simulink model "disturbances_test"  (R2016b)
settings: Solver=VariableStepAuto  StartTime=0.0  StopTime=5400  RelTol=1e-3
values from neighbouring files (symbols this model uses):
  fsw_params = init_fsw_params()    [init_disturbances_test.m]    (also in init_environment_test.m)
undefined symbols (not defined in the file or in its folder): sim_params
libraries: environment_lib x2, aerolibutil x2, vrlib x1, time_conversions_lib x1, eci_2_ecef_lib x1, sgp4_lib_fsw x1, teme_2_eci_lib x1
settings Model: Creator=taylorreynolds  LastModifiedBy=taylorreynolds

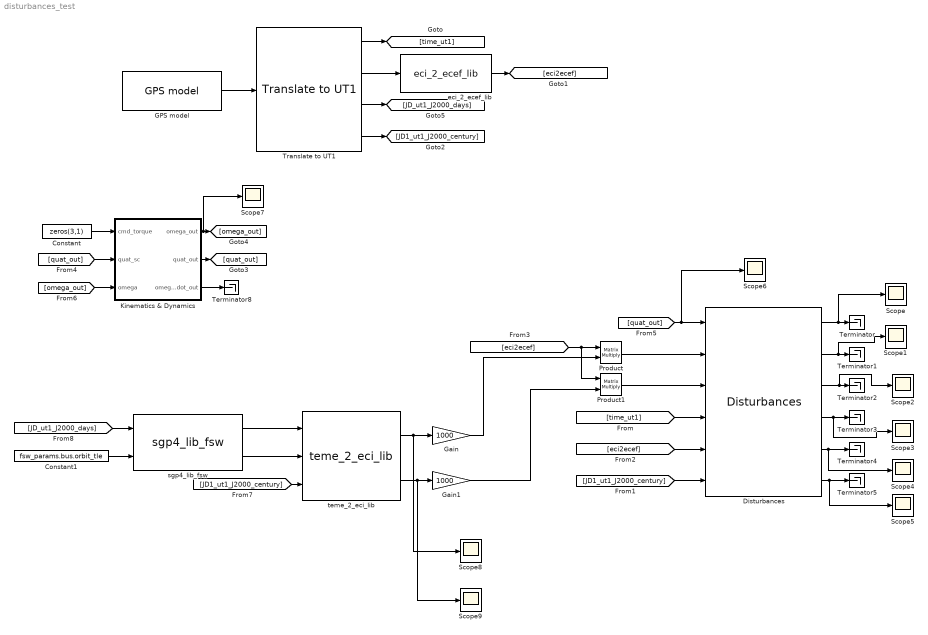
== system disturbances_test ==
  Constant : Constant  Value=zeros(3,1)
  Constant1 : Constant  Value=fsw_params.bus.orbit_tle
  Disturbances : environment_lib/Environment/Disturbances
  GPS model : environment_lib/Environment/GPS model
  Gain : Gain  Gain=1000
  Gain1 : Gain  Gain=1000
  Kinematics & Dynamics : Subsystem
  Product : Product  Multiplication=Matrix(*)
  Product1 : Product  Multiplication=Matrix(*)
  Scope{,1..9} (10 alike) : Scope
  Terminator{,1..5,8} (7 alike) : Terminator
  Translate to UT1 : time_conversions_lib/Translate to UT1
  eci_2_ecef_lib : eci_2_ecef_lib/eci_2_ecef_lib
  sgp4_lib_fsw : sgp4_lib_fsw/sgp4_lib_fsw
  teme_2_eci_lib : teme_2_eci_lib/teme_2_eci_lib
  wires:
  GPS model/1 -> Translate to UT1/1
  Translate to UT1/2 -> eci_2_ecef_lib/1
  Translate to UT1/1 -> [time_ut1]
  [time_ut1] -> Disturbances/4
  eci_2_ecef_lib/1 -> [eci2ecef]
  Translate to UT1/4 -> [JD1_ut1_J2000_century]
  [JD1_ut1_J2000_century] -> Disturbances/6
  [eci2ecef] -> Disturbances/5
  Gain/1 -> Product/2
  Product/1 -> Disturbances/2
  Product1/1 -> Disturbances/3
  Gain1/1 -> Product1/2
  [eci2ecef] -> Product1/1, Product/1
  Disturbances/1 -> Scope/1, Terminator/1
  Disturbances/2 -> Scope1/1, Terminator1/1
  Disturbances/3 -> Scope2/1, Terminator2/1
  Disturbances/4 -> Scope3/1, Terminator3/1
  Disturbances/5 -> Terminator4/1, Scope4/1
  Disturbances/6 -> Scope5/1, Terminator5/1
  Translate to UT1/3 -> [JD_ut1_J2000_days]
  Constant/1 -> Kinematics & Dynamics/1(cmd_torque)
  Kinematics & Dynamics/1(omega_out) -> Scope7/1, [omega_out]
  Kinematics & Dynamics/3(omega_dot_out) -> Terminator8/1
  Kinematics & Dynamics/2(quat_out) -> [quat_out]
  [quat_out] -> Scope6/1, Disturbances/1
  [quat_out] -> Kinematics & Dynamics/2(quat_sc)
  [omega_out] -> Kinematics & Dynamics/3(omega)
  Constant1/1 -> sgp4_lib_fsw/2
  teme_2_eci_lib/2 -> Scope9/1, Gain1/1
  teme_2_eci_lib/1 -> Scope8/1, Gain/1
  sgp4_lib_fsw/1 -> teme_2_eci_lib/1
  sgp4_lib_fsw/2 -> teme_2_eci_lib/2
  [JD1_ut1_J2000_century] -> teme_2_eci_lib/3
  [JD_ut1_J2000_days] -> sgp4_lib_fsw/1

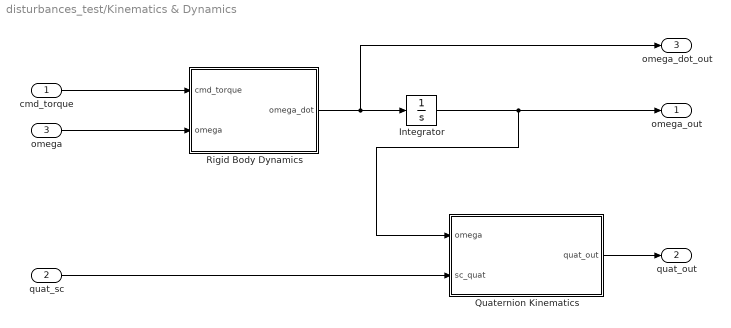
== system disturbances_test/Kinematics & Dynamics ==
  cmd_torque : Inport
  quat_sc : Inport  Port=2
  omega : Inport  Port=3
  Integrator : Integrator  InitialCondition=sim_params.dynamics.ic.rate_init
  Quaternion Kinematics : Subsystem
  Rigid Body Dynamics : Subsystem
  omega_out : Outport
  quat_out : Outport  Port=2
  omega_dot_out : Outport  Port=3
  wires:
  Rigid Body Dynamics/1(omega_dot) -> omega_dot_out/1, Integrator/1
  Integrator/1 -> Quaternion Kinematics/1(omega), omega_out/1
  cmd_torque/1 -> Rigid Body Dynamics/1(cmd_torque)
  omega/1 -> Rigid Body Dynamics/2(omega)
  Quaternion Kinematics/1(quat_out) -> quat_out/1
  quat_sc/1 -> Quaternion Kinematics/2(sc_quat)

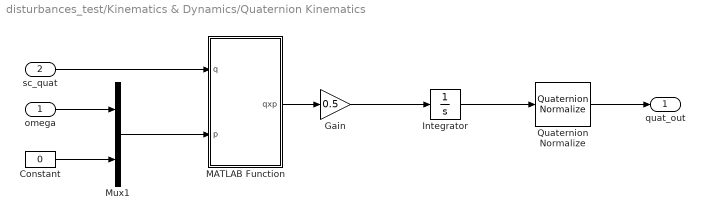
== system disturbances_test/Kinematics & Dynamics/Quaternion Kinematics ==
  omega : Inport
  sc_quat : Inport  Port=2
  Constant : Constant  Value=0
  Gain : Gain  Gain=0.5
  Integrator : Integrator  InitialCondition=sim_params.dynamics.ic.quat_init
  MATLAB Function : MATLAB Function  TreatAsAtomicUnit=on
  Mux1 : Mux  Inputs=[3 1]
  Quaternion Normalize : aerolibutil/Quaternion Normalize
  quat_out : Outport
  wires:
  Mux1/1 -> MATLAB Function/2(p)
  MATLAB Function/1(qxp) -> Gain/1
  Gain/1 -> Integrator/1
  Integrator/1 -> Quaternion Normalize/1
  Quaternion Normalize/1 -> quat_out/1
  sc_quat/1 -> MATLAB Function/1(q)
  omega/1 -> Mux1/1
  Constant/1 -> Mux1/2

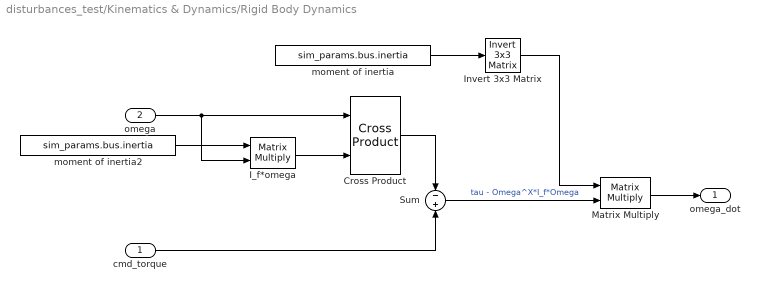
== system disturbances_test/Kinematics & Dynamics/Rigid Body Dynamics ==
  cmd_torque : Inport
  omega : Inport  Port=2
  Cross Product : vrlib/Utilities/Cross Product
  I_f*omega : Product  Multiplication=Matrix(*)
  Invert 3x3 Matrix : aerolibutil/Invert  3x3 Matrix
  "Matrix Multiply " : Product  Multiplication=Matrix(*)
  Sum : Sum  Inputs=-+
  moment of inertia : Constant  Value=sim_params.bus.inertia
  moment of inertia2 : Constant  Value=sim_params.bus.inertia
  omega_dot : Outport
  wires:
  omega/1 -> I_f*omega/2, Cross Product/1
  moment of inertia/1 -> Invert 3x3 Matrix/1
  I_f*omega/1 -> Cross Product/2
  cmd_torque/1 -> Sum/2
  Invert 3x3 Matrix/1 -> "Matrix Multiply "/1
  Sum/1 -> "Matrix Multiply "/2  "tau - Omega^X*I_f*Omega"
  "Matrix Multiply "/1 -> omega_dot/1
  Cross Product/1 -> Sum/1
  moment of inertia2/1 -> I_f*omega/1

== matlab function disturbances_test/Kinematics & Dynamics/Quaternion Kinematics/MATLAB Function ==
  data: q input; qxp output; p input
function qxp   = Q_mult( q,p )

% Multiplies two quaternions according to a SCALAR LAST convention.
% T. Reynolds, RAIN Lab, 8.2.17

if length(q) ~= 4 || length(p) ~= 4
    error('One of the input vectors is not a quaternion')
end

q   = reshape(q,4,1);
p   = reshape(p,4,1);

qv  = q(1:3);
q0  = q(4);
pv  = p(1:3);
p0  = p(4);

qxp_v   = p0*qv + q0*pv + skew(qv)*pv;
qxp_0   = q0*p0 - pv'*qv;

qxp     = [ qxp_v; qxp_0 ];


end
